simulink model "amplificatorZgomot"  (R2022b)
settings: Solver=VariableStepAuto  StartTime=0.0  StopTime=10.0  RelTol=1e-3
settings Model: Creator=mihai  LastModifiedBy=mihai

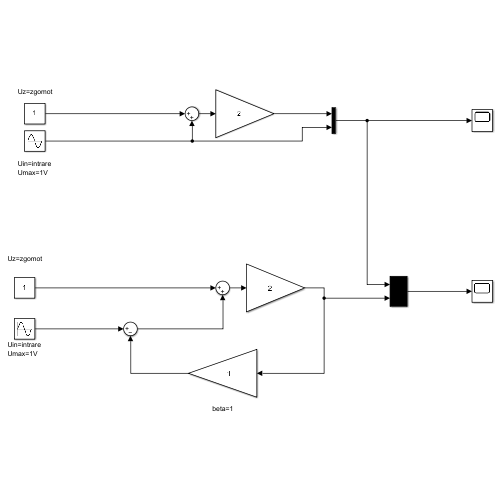
[thumbnail: Simulink's stored preview of the top-level diagram]
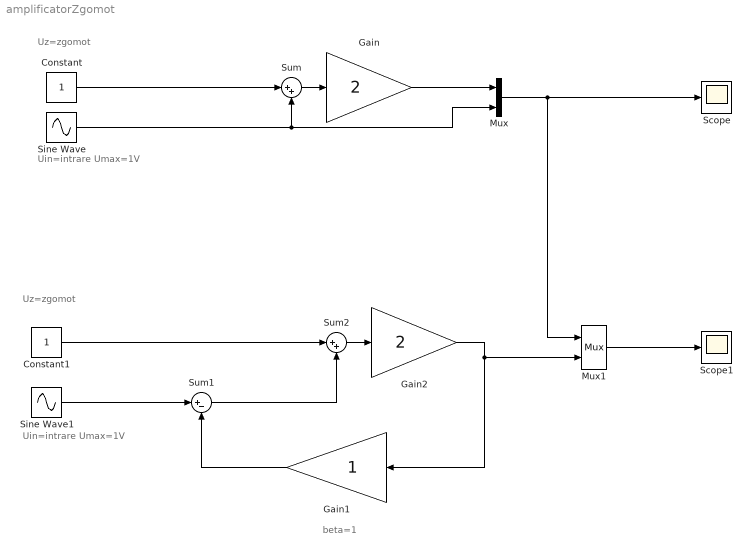
== system amplificatorZgomot ==
  note: beta=1
  note: Uin=intrare
      | Umax=1V
  note: Uz=zgomot
  note: Uin=intrare
      | Umax=1V
  note: Uz=zgomot
  Constant : Constant
  Constant1 : Constant
  Gain : Gain  Gain=2  SaturateOnIntegerOverflow=on  OutDataTypeStr=Inherit: Same as input  ParamDataTypeStr=Inherit: Same as input
  Gain1 : Gain  SaturateOnIntegerOverflow=on  OutDataTypeStr=Inherit: Same as input  ParamDataTypeStr=Inherit: Same as input
  Gain2 : Gain  Gain=2  SaturateOnIntegerOverflow=on  OutDataTypeStr=Inherit: Same as input  ParamDataTypeStr=Inherit: Same as input
  Mux : Mux  Inputs=2
  Mux1 : Mux  Inputs=2
  Scope : Scope
  Scope1 : Scope
  Sine Wave : Sin  SampleTime=0
  Sine Wave1 : Sin  SampleTime=0
  Sum : Sum  Inputs=|++
  Sum1 : Sum  Inputs=|+-
  Sum2 : Sum  Inputs=|++
  wires:
  Sine Wave/1 -> Sum/2, Mux/2
  Mux/1 -> Mux1/1, Scope/1
  Gain/1 -> Mux/1
  Sum/1 -> Gain/1
  Constant/1 -> Sum/1
  Mux1/1 -> Scope1/1
  Sum2/1 -> Gain2/1
  Gain2/1 -> Gain1/1, Mux1/2
  Constant1/1 -> Sum2/1
  Gain1/1 -> Sum1/2
  Sine Wave1/1 -> Sum1/1
  Sum1/1 -> Sum2/2
